simulink model "Quadcopter_01"  (R2021a)
settings: Solver=ode45  StartTime=0.0  StopTime=30  FixedStep=0.01  RelTol=1e-3
values from neighbouring files (symbols this model uses):
  x0 = [0;0;0;pi/3;0;0;0;0;0;0;0;0]    [Main_Simulation.m]
  xi0 = 0.1    [Main_Simulation.m]
  zeta0 = 0.1    [Main_Simulation.m]
settings Model: Creator=FawadFarooq  LastModifiedBy=FawadFarooq
settings DebuggingCC: UnderSpecifiedDimensionMsg=warning

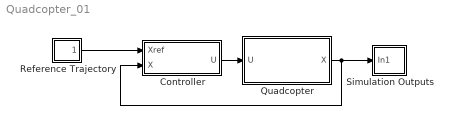
== system Quadcopter_01 ==
  Controller : Subsystem
  Quadcopter : Subsystem
  Reference Trajectory : Subsystem
  Simulation Outputs : Subsystem
  wires:
  Reference Trajectory/1(Xref) -> Controller/1(Xref)
  Quadcopter/1(X) -> Simulation Outputs/1(In1), Controller/2(X)
  Controller/1(U) -> Quadcopter/1(U)

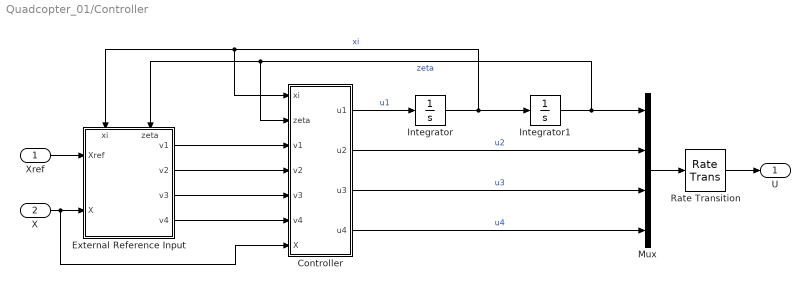
== system Quadcopter_01/Controller ==
  Xref : Inport
  X : Inport  Port=2
  Controller : MATLAB Function  TreatAsAtomicUnit=on
  External Reference Input : Subsystem
      settings: PortSchema="{\"entries\":[{\"content\":{\"sides\":[{\"content\":{\"connectorIds\":[\"In1\",\"In2\"]},\"type\":\"ConnectorPlacement.EquallySpacedRectSide\",\"uuid\":\"d1395934-ce6a-4464-9282-4ffb318fb487\"},{\"content\":{\"connectorIds\":[\"Out1\",\"Out2\",\"Out3\",\"Out4\"],\"side\":\"RIGHT\"},\"type\":\"ConnectorPlacement.EquallySpacedRectSide\",\"uuid\":\"caeb3e45-058f-47c8-bc51-7d909cb89f1f\"},{\"content\":{\"connectorIds\":[\"In3\",\"In4\"],\"side\":\"TOP\"},\"type\":\"ConnectorPlacement.EquallySpacedRectSide\",\"uuid\":\"43d47942-84b8-4468-9704-f3501b244f2e\"}]},\"type\":\"ConnectorPlacement.EquallySpacedConnector\",\"uuid\":\"77f035cc-3394-47d2-bba4-249502c9d3f6\"}],\"packageUris\":[\"http://schema.mathworks.com/mf0/Connector/R2020b\"],\"version\":\"1.0\"}"
  Integrator : Integrator  InitialCondition=zeta0
  Integrator1 : Integrator  InitialCondition=xi0
  Mux : Mux
  Rate Transition : RateTransition  OutPortSampleTime=0.01
  U : Outport
  wires:
  X/1 -> Controller/7(X), External Reference Input/2(X)
  Xref/1 -> External Reference Input/1(Xref)
  External Reference Input/1(v1) -> Controller/3(v1)
  External Reference Input/2(v2) -> Controller/4(v2)
  External Reference Input/3(v3) -> Controller/5(v3)
  External Reference Input/4(v4) -> Controller/6(v4)
  Controller/1(u1) -> Integrator/1  "u1"
  Controller/2(u2) -> Mux/2  "u2"
  Controller/3(u3) -> Mux/3  "u3"
  Controller/4(u4) -> Mux/4  "u4"
  Mux/1 -> Rate Transition/1
  Integrator/1 -> Controller/1(xi), External Reference Input/3(xi), Integrator1/1  "xi"
  Integrator1/1 -> Mux/1, Controller/2(zeta), External Reference Input/4(zeta)  "zeta"
  Rate Transition/1 -> U/1

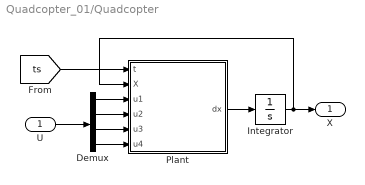
== system Quadcopter_01/Quadcopter ==
  U : Inport
  Demux : Demux
  Integrator : Integrator  InitialCondition=x0
  Plant : MATLAB Function  TreatAsAtomicUnit=on
  X : Outport
  wires:
  Plant/1(dx) -> Integrator/1
  [ts] -> Plant/1(t)
  U/1 -> Demux/1
  Integrator/1 -> Plant/2(X), X/1
  Demux/1 -> Plant/3(u1)
  Demux/2 -> Plant/4(u2)
  Demux/3 -> Plant/5(u3)
  Demux/4 -> Plant/6(u4)

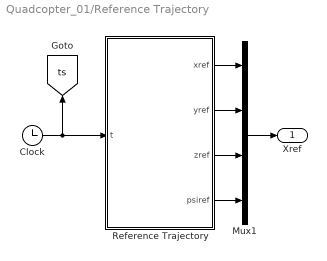
== system Quadcopter_01/Reference Trajectory ==
  Clock : Clock
  Mux1 : Mux
  Reference Trajectory : MATLAB Function  TreatAsAtomicUnit=on
  Xref : Outport
  tag scope: ts=global
  wires:
  Clock/1 -> Reference Trajectory/1(t), [ts]
  Reference Trajectory/1(xref) -> Mux1/1
  Reference Trajectory/2(yref) -> Mux1/2
  Reference Trajectory/3(zref) -> Mux1/3
  Reference Trajectory/4(psiref) -> Mux1/4
  Mux1/1 -> Xref/1

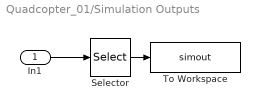
== system Quadcopter_01/Simulation Outputs ==
  In1 : Inport
  Selector : Selector  InputPortWidth=12  IndexOptions=Index vector (dialog)  Indices=[1,2,3]  OutputSizes=1
  To Workspace : ToWorkspace  VariableName=simout  SaveFormat=Timeseries  SampleTime=-1
  wires:
  Selector/1 -> To Workspace/1
  In1/1 -> Selector/1

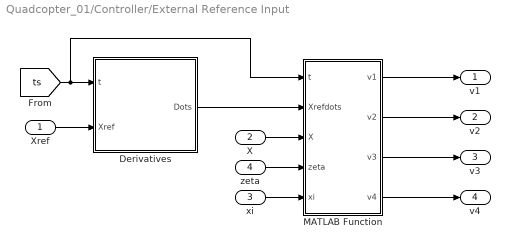
== system Quadcopter_01/Controller/External Reference Input ==
  Xref : Inport
  X : Inport  Port=2
  xi : Inport  Port=3
  zeta : Inport  Port=4
  Derivatives : Subsystem
  MATLAB Function : MATLAB Function  TreatAsAtomicUnit=on
  v1 : Outport
  v2 : Outport  Port=2
  v3 : Outport  Port=3
  v4 : Outport  Port=4
  wires:
  MATLAB Function/1(v1) -> v1/1
  MATLAB Function/2(v2) -> v2/1
  MATLAB Function/3(v3) -> v3/1
  MATLAB Function/4(v4) -> v4/1
  X/1 -> MATLAB Function/3(X)
  Xref/1 -> Derivatives/2(Xref)
  Derivatives/1(Dots) -> MATLAB Function/2(Xrefdots)
  zeta/1 -> MATLAB Function/4(zeta)
  xi/1 -> MATLAB Function/5(xi)
  [ts] -> MATLAB Function/1(t), Derivatives/1(t)

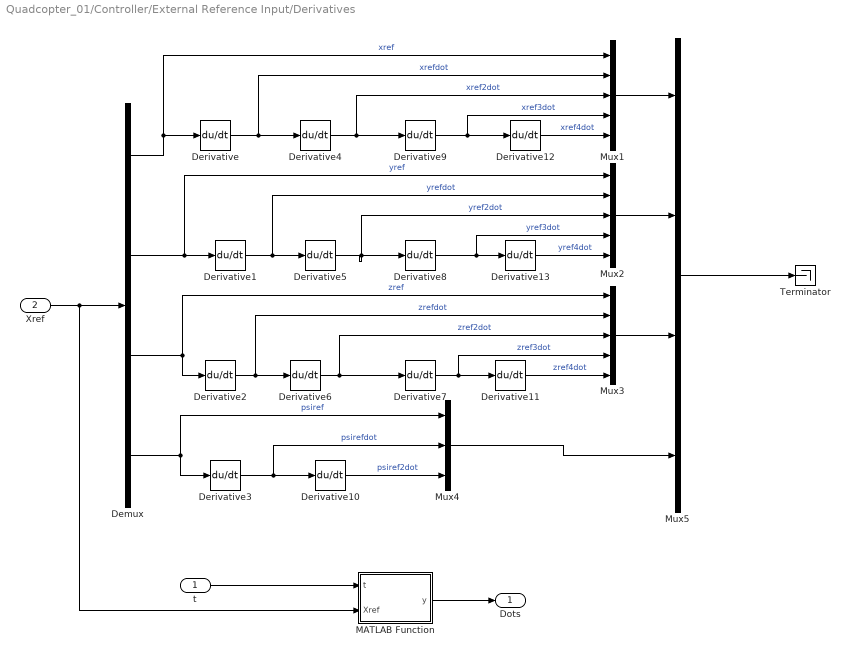
== system Quadcopter_01/Controller/External Reference Input/Derivatives ==
  t : Inport
  Xref : Inport  Port=2
  Demux : Demux
  Derivative{,1..13} (14 alike) : Derivative
  MATLAB Function : MATLAB Function  TreatAsAtomicUnit=on
  Mux1 : Mux  Inputs=5
  Mux2 : Mux  Inputs=5
  Mux3 : Mux  Inputs=5
  Mux4 : Mux  Inputs=3
  Mux5 : Mux
  Terminator : Terminator
  Dots : Outport
  wires:
  Derivative3/1 -> Mux4/2, Derivative10/1  "psirefdot"
  Derivative/1 -> Derivative4/1, Mux1/2  "xrefdot"
  Derivative5/1 -> Derivative8/1, Mux2/3  "yref2dot"
  Demux/1 -> Derivative/1, Mux1/1  "xref"
  Mux1/1 -> Mux5/1
  Derivative4/1 -> Mux1/3, Derivative9/1  "xref2dot"
  Demux/3 -> Derivative2/1, Mux3/1  "zref"
  Demux/2 -> Derivative1/1, Mux2/1  "yref"
  Xref/1 -> MATLAB Function/2(Xref), Demux/1
  Demux/4 -> Derivative3/1, Mux4/1  "psiref"
  Derivative2/1 -> Mux3/2, Derivative6/1  "zrefdot"
  Mux4/1 -> Mux5/4
  Derivative1/1 -> Derivative5/1, Mux2/2  "yrefdot"
  Mux3/1 -> Mux5/3
  Derivative6/1 -> Derivative7/1, Mux3/3  "zref2dot"
  Mux2/1 -> Mux5/2
  Derivative7/1 -> Mux3/4, Derivative11/1  "zref3dot"
  Derivative8/1 -> Mux2/4, Derivative13/1  "yref3dot"
  Derivative9/1 -> Derivative12/1, Mux1/4  "xref3dot"
  Derivative10/1 -> Mux4/3  "psiref2dot"
  Derivative11/1 -> Mux3/5  "zref4dot"
  Derivative12/1 -> Mux1/5  "xref4dot"
  Derivative13/1 -> Mux2/5  "yref4dot"
  Mux5/1 -> Terminator/1
  MATLAB Function/1(y) -> Dots/1
  t/1 -> MATLAB Function/1(t)

== matlab function Quadcopter_01/Reference Trajectory/Reference Trajectory ==
  data: t input; xref output; yref output; zref output; psiref output
function [xref,yref,zref,psiref] = fcn(t)

xref = 1/2*cos(t/2);

yref = 1/2*sin(t/2);

zref = 1+t/10;

psiref = pi/3;

== matlab function Quadcopter_01/Quadcopter/Plant ==
  data: t input; dx output; X input; u1 input; u2 input; u3 input; u4 input
function dx = fcn(t,X,u1,u2,u3,u4)

% Assigning States
x     = X(1);
y     = X(2);
z     = X(3);
psi   = X(4);
theta = X(5);
phi   = X(6);
u     = X(7);
v     = X(8);
w     = X(9);
p     = X(10);
q     = X(11);
r     = X(12);

% Constants
fp.T   = 0.01;
fp.m   = 0.7;
fp.l   = 0.3;
fp.Ixx = 1.2416;
fp.Iyy = 1.2416;
fp.Izz = 1.2416;
fp.g   = 9.81;

% Disturbances

d = [1;1;1];
if (t<5 || t>15);  d(1) = 0;end
if (t<8 || t>15);  d(2) = 0;end
if (t<10 || t>15); d(3) = 0;end

% Differential Equations

xdot     = u;
ydot     = v;
zdot     = w;
psidot   = q*sin(phi)*sec(theta) + r*cos(phi)*sec(theta);
thetadot = q*cos(phi) - r*sin(phi);
phidot   = p + q*sin(phi)*tan(theta) + r*cos(phi)*tan(theta);

% Remaining Differential Equations

udot     = d(1)/fp.m - u1*(1/fp.m)*(cos(psi)*sin(theta)*cos(phi) + sin(psi)*sin(phi));
vdot     = d(2)/fp.m - u1*(1/fp.m)*(sin(psi)*sin(theta)*cos(phi) - cos(psi)*sin(phi));
wdot     = d(3)/fp.m + fp.g - u1*(1/fp.m)*cos(theta)*cos(phi);

pdot     = (fp.Iyy-fp.Izz)/fp.Ixx*q*r + u2*fp.l/fp.Ixx;
qdot     = (fp.Izz-fp.Ixx)/fp.Iyy*p*r + u3*fp.l/fp.Iyy;
rdot     = (fp.Ixx-fp.Iyy)/fp.Izz*p*q + u4/fp.Izz;

dposition     = [xdot;ydot;zdot];
dvelocity     = [udot;vdot;wdot];
deuler_angles = [psidot;thetadot;phidot];
drates        = [pdot;qdot;rdot];

dx = [dposition;deuler_angles;dvelocity;drates];

== matlab function Quadcopter_01/Controller/Controller ==
  data: xi input; zeta input; v1 input; u1 output; v2 input; v3 input; v4 input; u2 output; u3 output; u4 output; X input
function [u1,u2,u3,u4] = fcn(xi,zeta,v1,v2,v3,v4,X)

x     = X(1);
y     = X(2);
z     = X(3);
psi   = X(4);
theta = X(5);
phi   = X(6);
u     = X(7);
v     = X(8);
w     = X(9);
p     = X(10);
q     = X(11);
r     = X(12);

%%

b = [(10*p^2*zeta*sin(phi)*sin(psi))/7 + (10*q^2*zeta*sin(phi)*sin(psi))/7 - (20*q*xi*cos(psi)*cos(theta))/7 - (20*p*xi*cos(phi)*sin(psi))/7 + (10*p^2*zeta*cos(phi)*cos(psi)*sin(theta))/7 + (10*q^2*zeta*cos(phi)*cos(psi)*sin(theta))/7 - (10*p*r*zeta*cos(psi)*cos(theta))/7 + (10*q*r*zeta*cos(phi)*sin(psi))/7 + (20*p*xi*cos(psi)*sin(phi)*sin(theta))/7 - (10*q*r*zeta*cos(psi)*sin(phi)*sin(theta))/7;
    (20*p*xi*cos(phi)*cos(psi))/7 - (10*p^2*zeta*cos(psi)*sin(phi))/7 - (10*q^2*zeta*cos(psi)*sin(phi))/7 - (20*q*xi*cos(theta)*sin(psi))/7 + (10*p^2*zeta*cos(phi)*sin(psi)*sin(theta))/7 + (10*q^2*zeta*cos(phi)*sin(psi)*sin(theta))/7 - (10*q*r*zeta*cos(phi)*cos(psi))/7 - (10*p*r*zeta*cos(theta)*sin(psi))/7 + (20*p*xi*sin(phi)*sin(psi)*sin(theta))/7 - (10*q*r*zeta*sin(phi)*sin(psi)*sin(theta))/7;
    (20*q*xi*sin(theta))/7 + (20*p*xi*cos(theta)*sin(phi))/7 + (10*p^2*zeta*cos(phi)*cos(theta))/7 + (10*q^2*zeta*cos(phi)*cos(theta))/7 + (10*p*r*zeta*sin(theta))/7 - (10*q*r*zeta*cos(theta)*sin(phi))/7;
    ((q*cos(phi) - r*sin(phi))*(p*cos(theta) + 2*r*cos(phi)*sin(theta) + 2*q*sin(phi)*sin(theta)))/cos(theta)^2];

deltaX = [
    [- (10*sin(phi)*sin(psi))/7 - (10*cos(phi)*cos(psi)*sin(theta))/7, (1875*zeta*cos(psi)*sin(phi)*sin(theta))/5432 - (1875*zeta*cos(phi)*sin(psi))/5432, -(1875*zeta*cos(psi)*cos(theta))/5432,                               0];
    [  (10*cos(psi)*sin(phi))/7 - (10*cos(phi)*sin(psi)*sin(theta))/7, (1875*zeta*cos(phi)*cos(psi))/5432 + (1875*zeta*sin(phi)*sin(psi)*sin(theta))/5432, -(1875*zeta*cos(theta)*sin(psi))/5432,                               0];
    [                                     -(10*cos(phi)*cos(theta))/7,                                               (1875*zeta*cos(theta)*sin(phi))/5432,           (1875*zeta*sin(theta))/5432,                               0];
    [                                                               0,                                                                                  0,      (375*sin(phi))/(1552*cos(theta)), (625*cos(phi))/(776*cos(theta))]
    ];

alpha = -inv(deltaX)*b;
beta  = inv(deltaX);


V = [v1;v2;v3;v4];

ubar = alpha + beta*V;

u1 = ubar(1);
u2 = ubar(2);
u3 = ubar(3);
u4 = ubar(4);

== matlab function Quadcopter_01/Controller/External Reference Input/MATLAB Function ==
  data: t input; Xrefdots input; v1 output; X input; v2 output; v3 output; v4 output; zeta input; xi input
function [v1,v2,v3,v4] = fcn(t,Xrefdots,X,zeta,xi)

[d1,d2,d3] = deal(1,1,1);
if (t<5 || t>15);  d1 = 0;end
if (t<8 || t>15);  d2 = 0;end
if (t<10 || t>15); d3 = 0;end

fp.c0  = 625;
fp.c1  = 500;
fp.c2  = 150;
fp.c3  = 20;
fp.c4  = 4;
fp.c5  = 4;

% Assign to Variables
xref     = Xrefdots(1);
xrefdot  = Xrefdots(2);
xref2dot = Xrefdots(3);
xref3dot = Xrefdots(4);
xref4dot = Xrefdots(5);

yref     = Xrefdots(6);
yrefdot  = Xrefdots(7);
yref2dot = Xrefdots(8);
yref3dot = Xrefdots(9);
yref4dot = Xrefdots(10);

zref     = Xrefdots(11);
zrefdot  = Xrefdots(12);
zref2dot = Xrefdots(13);
zref3dot = Xrefdots(14);
zref4dot = Xrefdots(15);

psiref     = Xrefdots(16);
psirefdot  = Xrefdots(17);
psiref2dot = Xrefdots(18);

x     = X(1);
y     = X(2);
z     = X(3);
psi   = X(4);
theta = X(5);
phi   = X(6);
u     = X(7);
v     = X(8);
w     = X(9);
p     = X(10);
q     = X(11);
r     = X(12);

%%
xyzpsidot = [u;
    v;
    w;
    (r*cos(phi) + q*sin(phi))/cos(theta)];

xyz2dot = [(10*d1)/7 - zeta*((10*sin(phi)*sin(psi))/7 + (10*cos(phi)*cos(psi)*sin(theta))/7);
    (10*d2)/7 + zeta*((10*cos(psi)*sin(phi))/7 - (10*cos(phi)*sin(psi)*sin(theta))/7);
    (10*d3)/7 - (10*zeta*cos(phi)*cos(theta))/7 + 981/100];

xyz3dot = [(10*p*zeta*cos(psi)*sin(phi)*sin(theta))/7 - (10*p*zeta*cos(phi)*sin(psi))/7 - (10*xi*cos(phi)*cos(psi)*sin(theta))/7 - (10*q*zeta*cos(psi)*cos(theta))/7 - (10*xi*sin(phi)*sin(psi))/7;
    (10*xi*cos(psi)*sin(phi))/7 - (10*q*zeta*cos(theta)*sin(psi))/7 - (10*xi*cos(phi)*sin(psi)*sin(theta))/7 + (10*p*zeta*cos(phi)*cos(psi))/7 + (10*p*zeta*sin(phi)*sin(psi)*sin(theta))/7;
    (10*q*zeta*sin(theta))/7 - (10*xi*cos(phi)*cos(theta))/7 + (10*p*zeta*cos(theta)*sin(phi))/7];


v1 = xref4dot - ...
    fp.c3*(xyz3dot(1)   - xref3dot) - ...
    fp.c2*(xyz2dot(1)   - xref2dot) - ...
    fp.c1*(xyzpsidot(1) - xrefdot) - ...
    fp.c0*(X(1)         - xref);

v2 = yref4dot - ...
    fp.c3*(xyz3dot(2)   - yref3dot) - ...
    fp.c2*(xyz2dot(2)   - yref2dot) - ...
    fp.c1*(xyzpsidot(2) - yrefdot) - ...
    fp.c0*(X(2)         - yref);

v3 = zref4dot - ...
    fp.c3*(xyz3dot(3)   - zref3dot) - ...
    fp.c2*(xyz2dot(3)   - zref2dot) - ...
    fp.c1*(xyzpsidot(3) - zrefdot) - ...
    fp.c0*(X(3)         - zref);

v4 = psiref2dot - ...
    fp.c5*(xyzpsidot(4) - psirefdot) - ...
    fp.c4*(X(4)         - psiref);

== matlab function Quadcopter_01/Controller/External Reference Input/Derivatives/MATLAB Function ==
  data: t input; Xref input; y output
function y = fcn(t,Xref)

xref   = Xref(1);
yref   = Xref(2);
zref   = Xref(3);
psiref = Xref(4);

xrefdot  = sin(t./2.0).*(-1.0./4.0);
xref2dot = cos(t./2.0).*(-1.0./8.0);
xref3dot = sin(t./2.0)./1.6e+1;
xref4dot = cos(t./2.0)./3.2e+1;

yrefdot  = cos(t./2.0)./4.0;
yref2dot = sin(t./2.0).*(-1.0./8.0);
yref3dot = cos(t./2.0).*(-1.0./1.6e+1);
yref4dot = sin(t./2.0)./3.2e+1;

zrefdot  = 1.0./1.0e+1;
zref2dot = 0;
zref3dot = 0;
zref4dot = 0;

psirefdot  = 0;
psiref2dot = 0;

xrefD = [xref;xrefdot;xref2dot;xref3dot;xref4dot];
yrefD = [yref;yrefdot;yref2dot;yref3dot;yref4dot];
zrefD = [zref;zrefdot;zref2dot;zref3dot;zref4dot];
psirefD = [psiref;psirefdot;psiref2dot];

y = [xrefD;yrefD;zrefD;psirefD];
